simulink library "xps_library"  (Simulink 6.2)
values from neighbouring files (symbols this model uses):
  BEE2_ctrl =     [BEE2_hw_routes.mat]
  CORR =     [BEE2_hw_routes.mat]
  iBOB =     [BEE2_hw_routes.mat]
  out = 0    [read_xps.m]    (also in write_xps.m)
undefined symbols (not defined in the file or in its folder): powerpc405, xps_library_software_register_user_data_in
libraries: xbsIndex_r3 x302, simulink x29, dspsigops x12, xps_library x6
(part 1 of 3)
settings Model: LastModifiedBy=hchen05

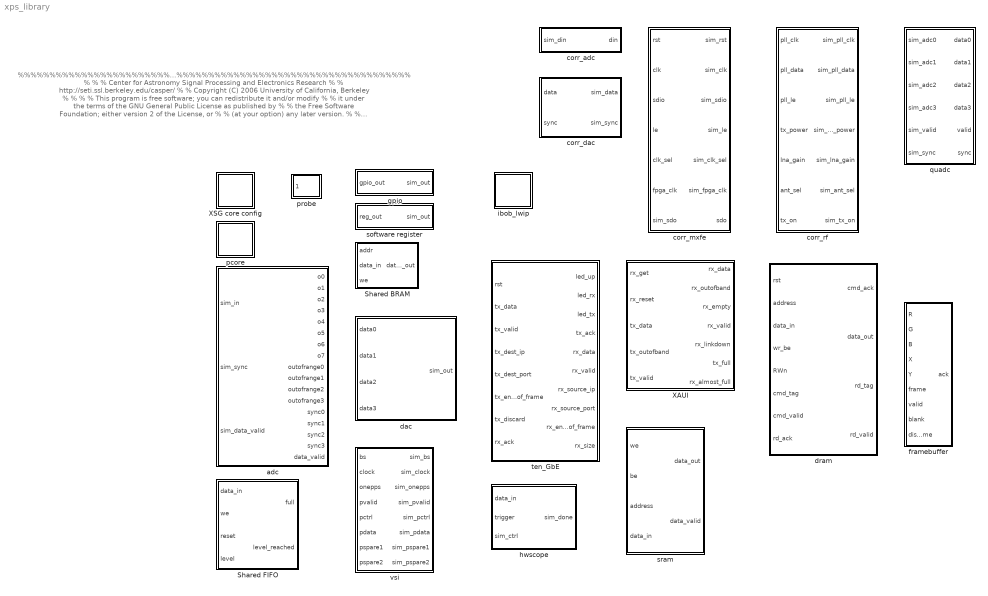
== system xps_library ==
  note: %%%%%%%%%%%%%%%%%%%%%%%%%%%%%%%%%%%%%%%%%%%%%%%%%%%%%%%%%%%%%%%%%%%%%%%%%%%%%%%
      | %                                                                             %
      | %   Center for Astronomy Signal Processing and Electronics Research           %
      | %   http://seti.ssl.berkeley.edu/casper/                                      %
      | %   Copyright (C) 2006 University of California, Berkeley                     %
      | %                                                                             %
      | %   This program is free software; you can redistribute it and/or modify      %
      | %   it under the terms of the GNU General Public License as published by      %
      | %   the Free Software Foundation; either version 2 of the License, or         %
      | %   (at your option) any later version.                                       %
      | %                                                                             %
      | %   This program is distributed in the hope that it will be useful,           %
      | %   but WITHOUT ANY WARRANTY; without even the implied warranty of            %
      | %   MERCHANTABILITY or FITNESS FOR A PARTICULAR PURPOSE.  See the             %
      | %   GNU General Public License for more details.                              %
      | %                                                                             %
      | %   You should have received a copy of the GNU General Public License along   %
      | %   with this program; if not, write to the Free Software Foundation, Inc.,   %
      | %   51 Franklin Street, Fifth Floor, Boston, MA 02110-1301 USA.               %
      | %                                                                             %
      | %%%%%%%%%%%%%%%%%%%%%%%%%%%%%%%%%%%%%%%%%%%%%%%%%%%%%%%%%%%%%%%%%%%%%%%%%%%%%%%
  Shared BRAM : Subsystem  Tag=xps:bram  mask{arith_type=Signed  (2's comp), addr_width=11, data_width=32, data_bin_pt=0, init_vals=[1:2^11], sample_rate=1}
      mask prompts: arith_type "Output Data Type"; addr_width "Address width"; data_width "Data Width"; data_bin_pt "Data Binary Point"; init_vals "Initial values (simulation only)"; sample_rate "Sample rate"
      mask init:
      | shared_bram_mask;
      mask StyleString: popup(Unsigned|Signed  (2's comp)),edit,edit,edit,edit,edit
  Shared FIFO : Subsystem  Tag=xps:fifo  mask{io_dir=To Processor, arith_type=Unsigned, data_width=32, data_bin_pt=0, fifo_length=512}
      mask prompts: io_dir "I/O Direction:"; arith_type "Data Type:"; data_width "Data Width:"; data_bin_pt "Data Binary Point:"; fifo_length "Depth:"
      mask init:
      | fifo_mask;
      mask StyleString: popup(From Processor|To Processor),popup(Unsigned|Signed  (2's comp)),popup(4|8|16|32|64|128|256),edit,popup(512|1024|2048|4096|8192|16384|32768|65536)
  XAUI : Subsystem  Tag=xps:xaui  mask(xaui){demux=1, port=iBOB:0, show_param=off, pre_emph=3, swing=800}
      mask prompts: show_param "---------------------- Show Implementation Parameters -----------------------------------------------------------------------------------"; pre_emph "Pre-emphasis"; swing "Differential swing"
      mask help: XAUI block for sending and receiving point-to-point, streaming data over the BEE2 and iBOB's CX4 connectors. NOTE: A new version of this block is in development.
      mask init:
      | xaui_mask;
      mask Help: eval('xlWeb([getenv(''MLIB_ROOT''), ''\doc\html\com_xaui\com_xaui.html''])')
      mask StyleString: popup(1|2),popup(iBOB:0|iBOB:1|BEE2_ctrl:0|BEE2_ctrl:1|BEE2_usr:0|BEE2_usr:1|BEE2_usr:2|BEE2_usr:3|CORR:0),checkbox,popup(0|1|2|3),popup(400|500|600|700|800)
      mask CallbackString:
      | ||myname=gcb;
      | if strcmp(get_param(myname, 'show_param'), 'on')
      |     set_param(myname, 'MaskVisibilities', {'on','on','on','on','on'});
      | else
      |     set_param(myname, 'MaskVisibilities', {'on','on','on','off','off'});
      | end||
  XSG core config : Subsystem  Tag=xps:xsg  mask(xsg core config){hw_sys=iBOB, ibob_linux=off, clk_src=sys_clk, gpio_clk_io_group=iBOB:sma, gpio_clk_bit_index=0, clk_rate=100, sample_period=1, synthesis_tool=XST, mpc_type=powerpc405}
      mask prompts: hw_sys "Hardware Platform"; ibob_linux "Include Linux add-on board support"; clk_src "User IP Clock source"; gpio_clk_io_group "GPIO Clock Pin I/O group"; gpio_clk_bit_index "GPIO Clock Pin bit index"; clk_rate "User IP Clock Rate (MHz)"; sample_period "Sample Period"; synthesis_tool "Synthesis Tool:"; mpc_type "Mask Parameter 10:"
      mask help:
      | The XSG Core Config block is used to configure the System Generator design
      | for the bee_xps toolflow. Settings here are used to configure the
      | Xilinx System Generator block parameters automatically, and control toolflow
      | script  execution. It needs to be at the top level of all designs being compiled
      | with the bee_xps toolflow.
      mask init:
      | xps_xsg_conf_mask;
      mask Help: eval('xlWeb([getenv(''MLIB_ROOT''), ''\doc\html\sys_xsg_core_config\sys_xsg_core_config.html''])')
      mask StyleString: popup(iBOB|BEE2_ctrl|BEE2_usr|CORR),checkbox,popup(sys_clk|sys_clk2x|usr_clk|usr_clk2x|adc0_clk|adc1_clk|dac0_clk|dac1_clk),popup(iBOB:gpio0|iBOB:gpio1|iBOB:gpio2|iBOB:gpio3|iBOB:sma|iBOB:zdok0|iBOB:zdok1|iBOB:mdr),edit,edit,edit,popup(Leonardo Spectrum|Synplify|Synplify Pro|XST),edit
      mask CallbackString:
      | myname=gcb;
      | if strcmp(get_param(myname,'hw_sys'), 'iBOB')
      |     if strmatch('usr_clk', get_param(myname,'clk_src'))
      |         set_param(myname, 'MaskVisibilities', {'on','on','on','on','on','on','on','on','off'});
      |     else
      |         set_param(myname, 'MaskVisibilities', {'on','on','on','off','off','on','on','on','off'});
      |     end
      | else
      |     set_param(myname, 'MaskVisibilities', {'on','off','on','off','off','on','on','on','off'});
      | end||myname=gcb;
      | if strcmp(get_param(myname,'hw_sys'), 'iBOB')
      |     if strmatch('usr_clk', get_param(myname,'clk_src'))
      |         set_param(myname, 'MaskVisibilities', {'on','on','on','on','on','on','on','on','off'});
      |     else
      |         set_param(myname, 'MaskVisibilities', {'on','on','on','off','off','on','on','on','off'});
      |     end
      | else
      |     set_param(myname, 'MaskVisibilities', {'on','off','on','off','off','on','on','on','off'});
      | end||||||
      mask Display: fprintf('MSSGE');
  adc : Subsystem  Tag=xps:adc  mask(adc){adc_brd=iBOB:adc0, adc_clk_rate=800, adc_interleave=on, sample_period=1}
      mask prompts: adc_brd "ADC board"; adc_clk_rate "ADC clock rate (MHz)"; adc_interleave "ADC interleave mode"; sample_period "Sample period"
      mask help: The ADC block converts analog inputs to digital outputs. Every clock cycle, the inputs are sampled and digitized to 8 bit binary point numbers in the range of [-1, 1) and are then output by the adc.
      mask init:
      | adc_mask;
      mask Help: eval('xlWeb([getenv(''MLIB_ROOT''), ''\doc\html\sys_adc\sys_adc.html''])')
      mask StyleString: popup(iBOB:adc0|iBOB:adc1),edit,checkbox,edit
  corr_adc : Subsystem  Tag=xps:corr_adc  mask{adc_brd=CORR:adc_i, arith_type=Signed  (2's comp), data_bin_pt=11, reg_clk_phase=0, sample_period=1}
      mask prompts: adc_brd "ADC:"; arith_type "Data type:"; data_bin_pt "Binary point:"; reg_clk_phase "Input sample clock phase:"; sample_period "Sample period:"
      mask init:
      | corr_adc_mask;
      mask StyleString: popup(CORR:adc_i|CORR:adc_q),popup(Unsigned|Signed  (2's comp)),edit,popup(0|90|180|270),edit
  corr_dac : Subsystem  Tag=xps:corr_dac  mask{arith_type=Unsigned, bin_pt=12, reg_clk_phase=0, sample_period=1}
      mask prompts: arith_type "Data Type:"; bin_pt "Data binary point (14-bit data):"; reg_clk_phase "Output sample clock phase:"; sample_period "Sample period:"
      mask init:
      | corr_dac_mask;
      mask StyleString: popup(Boolean|Unsigned|Signed  (2's comp)),edit,popup(0|90|180|270),edit
  corr_mxfe : Subsystem  Tag=xps:corr_mxfe  mask{reg_clk_phase=0, sample_period=1}
      mask prompts: reg_clk_phase "Input sample clock phase:"; sample_period "Sample period:"
      mask init:
      | corr_mxfe_mask;
      mask StyleString: popup(0|90|180|270),edit
  corr_rf : Subsystem  Tag=xps:corr_rf  mask{arith_type=Unsigned, bin_pt=0, sample_period=1}
      mask prompts: arith_type "TX power data type:"; bin_pt "TX power binary point (3-bit data):"; sample_period "Sample period:"
      mask init:
      | corr_rf_mask;
      mask StyleString: popup(Boolean|Unsigned|Signed  (2's comp)),edit,edit
  dac : Subsystem  Tag=xps:dac  mask(dac){dac_brd=iBOB:dac0, dac_clk_rate=800, sample_period=1, show_param=off, invert_clock=off}
      mask prompts: dac_brd "DAC board"; dac_clk_rate "DAC clock rate (MHz)"; sample_period "Sample period"; show_param "---------------------- Show Implementation Parameters -----------------------------------------------------------------------------------"; invert_clock "Invert output clock phase"
      mask help: Interface to SiBeam single Atmel TS86101G2B DAC board. The DAC block converts 4 digital inputs to 1 analog output. The dac runs at 4x FPGA clock frequency, outputting analog converted samples 0 through 3 each FPGA clock cycle.
      mask init:
      | dac_mask;
      mask Help: eval('xlWeb([getenv(''MLIB_ROOT''), ''\doc\html\sys_dac\sys_dac.html''])')
      mask StyleString: popup(iBOB:dac0|iBOB:dac1),edit,edit,checkbox,checkbox
      mask CallbackString:
      | |||myname=gcb;
      | if strcmp(get_param(myname, 'show_param'), 'on')
      |     set_param(myname, 'MaskVisibilities', {'on','on','on','on','on'});
      | else
      |     set_param(myname, 'MaskVisibilities', {'on','on','on','on','off'});
      | end|
  dram : Subsystem  Tag=xps:dram  mask(dram){dimm=1, arith_type=Unsigned, bin_pt=0, ip_clock=200, sample_period=1, use_sim=on, bank_mgt=off, wide_data=off, half_burst=off}
      mask prompts: arith_type "Data Type"; bin_pt "Data binary point"; ip_clock "Datapath clock rate (MHz)"; sample_period "Sample period"; use_sim "Simulate DRAM using ModelSim"; bank_mgt "Enable bank management"; wide_data "Use wide data bus (288 bits)"; half_burst "Use half-burst"
      mask help:
      | Interface to 1GB DDR2 DIMMs on BEE2.
      |
      | To simulate using ModelSim, place a ModelSim block named 'ModelSim' (case-sensitive) in the top level of the design.
      |
      | Commands that are clocked-in are executed with an unknown delay, however, execution order is maintained.
      mask init:
      | dram_mask;
      mask Help: eval('xlWeb([getenv(''MLIB_ROOT''), ''\doc\html\sys_dram\sys_dram.html''])')
      mask StyleString: popup(1|2|3|4),popup(Boolean|Unsigned|Signed  (2's comp)),edit,edit,edit,checkbox,checkbox,checkbox,checkbox
      mask CallbackString:
      | |||||||myname=gcb;
      | if strcmp(get_param(myname, 'wide_data'), 'off')
      |     set_param(myname, 'MaskEnables', {'on','on','on','on','on','on','on','on','on'});
      | else
      |     set_param(myname, 'half_burst', 'off');
      |     set_param(myname, 'MaskEnables', {'on','on','on','on','on','on','on','on','off'});
      | end|
  framebuffer : Subsystem  Tag=xps:framebuffer  mask(framebuffer){dimm=2, sample_period=1}
      mask prompts: sample_period "Sample period"
      mask help: Interface to Framebuffer.
      mask init:
      | framebuffer_mask;
      mask StyleString: popup(2|3|4),edit
  gpio : Subsystem  Tag=xps:gpio  mask(gpio){io_group=iBOB:led, io_dir=out, arith_type=Boolean, bitwidth=1, bin_pt=0, bit_index=0, sample_period=1, use_single_ended=off, use_ddr=off, reg_iob=on, reg_clk_phase=0, termination=None}
      mask prompts: io_group "I/O group"; io_dir "I/O direction"; arith_type "Data Type"; bitwidth "Data bitwidth"; bin_pt "Data binary point"; bit_index "GPIO bit index"; sample_period "Sample period"; use_single_ended "Use as single-ended"; use_ddr "Use DDR"; reg_iob "Pack register in the pad"; reg_clk_phase "Register clock phase"; termination "Termination method"
      mask help: GPIO interfaces for BEE2, iBOB, and CORR boards.
      mask init:
      | gpio_mask;
      mask StyleString: popup(iBOB:led|iBOB:dipsw|iBOB:gpio0|iBOB:gpio1|iBOB:gpio2|iBOB:gpio3|iBOB:zdok0|iBOB:zdok1|iBOB:mdr|iBOB:sma|BEE2_ctrl:led|BEE2_ctrl:downlink1|BEE2_ctrl:downlink2|BEE2_ctrl:downlink3|BEE2_ctrl:downlink4|BEE2_usr:led|BEE2_usr:gpio|BEE2_usr:bus_ctrl|BEE2_usr:bus_data|BEE2_usr:uplink|BEE2_usr:leftlink|BEE2_usr:rightlink|CORR:four_buttons|CORR:six_buttons|CORR:led|CORR:jumper_driver|CORR:jumper_receiver),popup(in|out),popup(Boolean|Unsigned|Signed  (2's comp)),edit,edit,edit,edit,checkbox,checkbox,checkbox,popup(0|90|180|270),popup(None|Pullup|Pulldown)
      mask CallbackString:
      | if ~isempty(find(strcmp(get_param(gcb, 'io_group'), {'iBOB:zdok0' 'iBOB:zdok1' 'iBOB:mdr'})))
      |     set_param(gcb, 'MaskVisibilities', {'on','on','on','on','on','on','on','on','on','on','on','on'});
      | else
      |     set_param(gcb, 'MaskVisibilities', {'on','on','on','on','on','on','on','off','on','on','on','on'});
      | end|||||||if ~isempty(find(strcmp(get_param(gcb,'io_group'),{'iBOB:zdok0','iBOB:zdok1','iBOB:mdr'}))) & strcmp(get_param(gcb,'use_single_ended'),'on')
      |     warndlg('The selected I/O group is routed as a differential pair on the board. Using these I/Os in single-ended mode may degrade signal integrity performance.')
      | end|if strcmp(get_param(gcb,'use_ddr'),'on')
      |     set_param(gcb,'reg_iob','on');
      | end|||
  hwscope : Subsystem  mask{scope_depth=2048, sim_trig_delay=8}
      mask prompts: scope_depth "Scope depth:"; sim_trig_delay "Trigger delay (simulation only):"
      mask init:
      | cursys = gcb;
      | set_param([cursys,'/scopefifo'], 'fifo_length', scope_depth);
      mask StyleString: popup(512|1024|2048|4096|8192|16384|32768|65536),edit
  ibob_lwip : Subsystem
      mask Type: ibobethlite
      mask Description: Attaches SRAM0 to the PLB bus and adds LWIP support.
      mask Display: fprintf('IBOB\nLWIP');
  pcore : Subsystem  Tag=xps:pcore  mask(pcore){pcore_path=customlib/pcores}
      mask prompts: pcore_path "Custom pcores path"
      mask help: Allows insertion of custom EDK pcores not distributed with base systems.
      mask Display: fprintf('PCORE');
  probe : Subsystem  Tag=xps:probe  mask{ila_number=0, match_type=basic, match_counter_width=8, capture_depth=512, arith_type=Boolean, bitwidth=1, bin_pt=0}
      mask prompts: ila_number "Chipscope ILA number"; match_type "Match Unit Type"; match_counter_width "Match counter width"; capture_depth "Probe capture depth"; arith_type "Data type"; bitwidth "Data bit width"; bin_pt "Data binary point"
      mask init:
      | probe_mask;
      mask StyleString: popup(0|1|2|3|4|5|6|7|8|9|10|11|12|13|14),popup(basic|basic with edges|extended|extended with edges|range|range with edges),popup(0|8|16|24|32),popup(512|1024|2048|4096|8192|16384),popup(Boolean|Unsigned|Signed  (2's comp)),edit,edit
  quadc : Subsystem  Tag=xps:quadc  mask(CASPER QuADC Interface Block){adc_brd=0, adc_clk_rate=200}
      mask prompts: adc_brd "ADC Board"; adc_clk_rate "ADC Clock Rate (MHz)"
      mask help: Interface block for the CASPER Quad ADC board (ADC4x250-8).
      mask init:
      | quadc_mask;
      mask StyleString: popup(0|1),edit
  software register : Subsystem  Tag=xps:sw_reg  mask{io_dir=To Processor, arith_type=Unsigned, bitwidth=32, bin_pt=0, sample_period=1, gw_name=xps_library_software_register_user_data_in}
      mask prompts: io_dir "I/O direction"; arith_type "Data Type"; bitwidth "Data bitwidth"; bin_pt "Data binary point"; sample_period "Sample period"; gw_name "Mask Parameter 6:"
      mask init:
      | register_mask;
      mask StyleString: popup(From Processor|To Processor),popup(Unsigned|Signed  (2's comp)),edit,edit,edit,edit
  sram : Subsystem  Tag=xps:sram  mask(sram){sram=0, arith_type=Unsigned, bin_pt=0, sample_period=1, use_sim=off}
      mask prompts: arith_type "Data Type"; bin_pt "Data binary point (bitwidth is 36)"; sample_period "Sample period"; use_sim "Simulate SRAM using ModelSim"
      mask help:
      | Interface to CY7C1370DV25 36x512k SRAMs on IBOB.
      |
      | To simulate using ModelSim, place a ModelSim block named 'ModelSim' (case-sensitive) in the top level of the design.
      |
      | The sram block represents a 36x512k SRAM chip on the IBOB. It stores 36-bit words and requires 19 bits to access its address space.
      mask init:
      | sram_mask;
      mask Help: eval('xlWeb([getenv(''MLIB_ROOT''), ''\doc\html\sys_sram\sys_sram.html''])')
      mask StyleString: popup(0|1),popup(Boolean|Unsigned|Signed  (2's comp)),edit,edit,checkbox
  ten_GbE : Subsystem  Tag=xps:tengbe  mask(ten_GbE){port=BEE2_ctrl:0, mac_lite=off, show_param=off, pre_emph=3, swing=800}
      mask prompts: mac_lite "Use light-weight MAC: Warning --> it DOES NOT check any CRC on receive"; show_param "---------------------- Show Implementation Parameters -----------------------------------------------------------------------------------"; pre_emph "Pre-emphasis"; swing "Differential swing"
      mask help: This block sends and receives UDP frames (packets). It accepts a 64 bit wide data stream with user-determined frame breaks. The data stream is wrapped in a UDP frame for transmission. Incoming UDP packets are unwrapped and the data presented as a 64 bit wide stream.
      mask init:
      | tengbe_mask;
      mask Help: eval('xlWeb([getenv(''MLIB_ROOT''), ''\doc\html\com_ten_GbE\com_ten_GbE.html''])')
      mask StyleString: popup(iBOB:0|iBOB:1|BEE2_ctrl:0|BEE2_ctrl:1|BEE2_usr:0|BEE2_usr:1|BEE2_usr:2|BEE2_usr:3|CORR:0),checkbox,checkbox,popup(0|1|2|3),popup(400|500|600|700|800)
      mask CallbackString:
      | ||myname=gcb;
      | if strcmp(get_param(myname, 'show_param'), 'on')
      |     set_param(myname, 'MaskVisibilities', {'on','on','on','on', 'on'});
      | else
      |     set_param(myname, 'MaskVisibilities', {'on','on','on','off','off'});
      | end||
  vsi : Subsystem  Tag=xps:vsi  mask(vsi){connector=MDR, arith_type=Unsigned, bin_pt=0, sample_period=1}
      mask prompts: arith_type "Data Type"; bin_pt "Data binary point (bitwidth is 32)"; sample_period "Sample period"
      mask help: Interface to MDR-80 connector on IBOB as configured for VLBI Standard Interface.
      mask init:
      | vsi_mask;
      mask StyleString: popup(MDR|ZDOK 1),popup(Boolean|Unsigned|Signed  (2's comp)),edit,edit

== system xps_library/Shared BRAM ==
  addr : Inport  Port=1  LatchInput=off
  data_in : Inport  Port=2  LatchInput=off
  we : Inport  Port=3  LatchInput=off
  Convert : xbsIndex_r3/Convert  arith_type=Unsigned  n_bits=addr_width  bin_pt=0  quantization=Truncate  overflow=Wrap  latency=0  explicit_period=off  period=1  dbl_ovrd=off  show_param=off  inserted_by_tool=off  pipeline=off
      settings: xl_area=[0, 0, 0, 0, 0, 0, 0]
  Convert1 : xbsIndex_r3/Convert  arith_type=Unsigned  n_bits=1  bin_pt=0  quantization=Truncate  overflow=Wrap  latency=0  explicit_period=off  period=1  dbl_ovrd=off  show_param=off  inserted_by_tool=off  pipeline=off
      settings: xl_area=[0, 0, 0, 0, 0, 0, 0]
  Convert2 : xbsIndex_r3/Convert  arith_type="Signed  (2's comp)"  n_bits=data_width  bin_pt=data_bin_pt  quantization=Truncate  overflow=Wrap  latency=0  explicit_period=off  period=1  dbl_ovrd=off  show_param=off  inserted_by_tool=off  pipeline=off
      settings: xl_area=[0, 0, 0, 0, 0, 0, 0]
  mem : Subsystem
  xps_library_Shared_BRAM_addr : xbsIndex_r3/Gateway Out  output_type=Double  nbits=8  bin_pt=6  arith_type=Boolean  quantization=Truncate  overflow=Wrap  hdl_port=on  timing_constraint=None  locs_specified=off  LOCs={'A5','B9','A9','C1','A3','G6','E9','A6','A7','A8','B8','B1','B3','D9','B5','B4','B6','C2'}  needs_fixed_name=on  show_param=off
      settings: xl_area=[0, 0, 0, 0, 0, 0, 0]
  xps_library_Shared_BRAM_data_in : xbsIndex_r3/Gateway Out  output_type=Double  nbits=8  bin_pt=6  arith_type=Boolean  quantization=Truncate  overflow=Wrap  hdl_port=on  timing_constraint=None  locs_specified=off  LOCs={'B21','B22','A22','B23','B19','C19','A20','A21','A23','B24','A24','A25','E18','D18','C18','B18'}  needs_fixed_name=on  show_param=off
      settings: xl_area=[0, 0, 0, 0, 0, 0, 0]
  xps_library_Shared_BRAM_data_out : xbsIndex_r3/Gateway In  arith_type="Signed  (2's comp)"  n_bits=data_width  bin_pt=data_bin_pt  quantization=Truncate  overflow=Wrap  period=sample_rate  timing_constraint=None  locs_specified=off  LOCs={}  needs_fixed_name=on  dbl_ovrd=off  show_param=off
      settings: xl_area=[0, 0, 0, 0, 0, 0, 0]
  xps_library_Shared_BRAM_we : xbsIndex_r3/Gateway Out  output_type=Double  nbits=8  bin_pt=6  arith_type=Boolean  quantization=Truncate  overflow=Wrap  hdl_port=on  timing_constraint=None  locs_specified=off  LOCs={'A14'}  needs_fixed_name=on  show_param=off
      settings: xl_area=[0, 0, 0, 0, 0, 0, 0]
  data_out : Outport
  wires:
  mem/1(Out1) -> xps_library_Shared_BRAM_data_out/1
  data_in/1 -> Convert2/1
  xps_library_Shared_BRAM_data_out/1 -> data_out/1
  addr/1 -> Convert/1
  we/1 -> Convert1/1
  Convert/1 -> xps_library_Shared_BRAM_addr/1
  Convert1/1 -> xps_library_Shared_BRAM_we/1
  Convert2/1 -> xps_library_Shared_BRAM_data_in/1
  xps_library_Shared_BRAM_addr/1 -> mem/1(In1)
  xps_library_Shared_BRAM_data_in/1 -> mem/2(In2)
  xps_library_Shared_BRAM_we/1 -> mem/3(In3)

== system xps_library/Shared FIFO ==
  data_in : Inport  Port=1  LatchInput=off
  we : Inport  Port=2  LatchInput=off
  reset : Inport  Port=3  LatchInput=off
  level : Inport  Port=4  LatchInput=off
  convert_xps_library_Shared_FIFO_user_data_in : xbsIndex_r3/Convert  arith_type=Unsigned  n_bits=32  bin_pt=0  quantization=Truncate  overflow=Wrap  latency=0  explicit_period=off  period=1  dbl_ovrd=off  show_param=off  inserted_by_tool=off  pipeline=off
      settings: xl_area=[0, 0, 0, 0, 0, 0, 0]
  convert_xps_library_Shared_FIFO_user_level : xbsIndex_r3/Convert  arith_type=Unsigned  n_bits=16  bin_pt=0  quantization=Truncate  overflow=Wrap  latency=0  explicit_period=off  period=1  dbl_ovrd=off  show_param=off  inserted_by_tool=off  pipeline=off
      settings: xl_area=[0, 0, 0, 0, 0, 0, 0]
  convert_xps_library_Shared_FIFO_user_reset : xbsIndex_r3/Convert  arith_type=Unsigned  n_bits=1  bin_pt=0  quantization=Truncate  overflow=Wrap  latency=0  explicit_period=off  period=1  dbl_ovrd=off  show_param=off  inserted_by_tool=off  pipeline=off
      settings: xl_area=[0, 0, 0, 0, 0, 0, 0]
  convert_xps_library_Shared_FIFO_user_we : xbsIndex_r3/Convert  arith_type=Unsigned  n_bits=1  bin_pt=0  quantization=Truncate  overflow=Wrap  latency=0  explicit_period=off  period=1  dbl_ovrd=off  show_param=off  inserted_by_tool=off  pipeline=off
      settings: xl_area=[0, 0, 0, 0, 0, 0, 0]
  xps_library_Shared_FIFO_user_data_in : xbsIndex_r3/Gateway Out  output_type=Double  nbits=8  bin_pt=6  arith_type=Boolean  quantization=Truncate  overflow=Wrap  hdl_port=on  timing_constraint=None  locs_specified=off  LOCs={}  needs_fixed_name=off  show_param=off
      settings: xl_area=[0, 0, 0, 0, 0, 0, 0]
  xps_library_Shared_FIFO_user_full : xbsIndex_r3/Gateway In  arith_type=Boolean  n_bits=1  bin_pt=0  quantization=Truncate  overflow=Wrap  period=1  timing_constraint=None  locs_specified=off  LOCs={}  needs_fixed_name=off  dbl_ovrd=off  show_param=off
      settings: xl_area=[0, 0, 0, 0, 0, 0, 0]
  xps_library_Shared_FIFO_user_level : xbsIndex_r3/Gateway Out  output_type=Double  nbits=8  bin_pt=6  arith_type=Boolean  quantization=Truncate  overflow=Wrap  hdl_port=on  timing_constraint=None  locs_specified=off  LOCs={}  needs_fixed_name=off  show_param=off
      settings: xl_area=[0, 0, 0, 0, 0, 0, 0]
  xps_library_Shared_FIFO_user_level_reached : xbsIndex_r3/Gateway In  arith_type=Boolean  n_bits=1  bin_pt=0  quantization=Truncate  overflow=Wrap  period=1  timing_constraint=None  locs_specified=off  LOCs={}  needs_fixed_name=off  dbl_ovrd=off  show_param=off
      settings: xl_area=[0, 0, 0, 0, 0, 0, 0]
  xps_library_Shared_FIFO_user_reset : xbsIndex_r3/Gateway Out  output_type=Double  nbits=8  bin_pt=6  arith_type=Boolean  quantization=Truncate  overflow=Wrap  hdl_port=on  timing_constraint=None  locs_specified=off  LOCs={}  needs_fixed_name=off  show_param=off
      settings: xl_area=[0, 0, 0, 0, 0, 0, 0]
  xps_library_Shared_FIFO_user_we : xbsIndex_r3/Gateway Out  output_type=Double  nbits=8  bin_pt=6  arith_type=Boolean  quantization=Truncate  overflow=Wrap  hdl_port=on  timing_constraint=None  locs_specified=off  LOCs={}  needs_fixed_name=off  show_param=off
      settings: xl_area=[0, 0, 0, 0, 0, 0, 0]
  full : Outport
  level_reached : Outport  Port=2
  wires:
  data_in/1 -> convert_xps_library_Shared_FIFO_user_data_in/1
  convert_xps_library_Shared_FIFO_user_data_in/1 -> xps_library_Shared_FIFO_user_data_in/1
  we/1 -> convert_xps_library_Shared_FIFO_user_we/1
  convert_xps_library_Shared_FIFO_user_we/1 -> xps_library_Shared_FIFO_user_we/1
  reset/1 -> convert_xps_library_Shared_FIFO_user_reset/1
  convert_xps_library_Shared_FIFO_user_reset/1 -> xps_library_Shared_FIFO_user_reset/1
  level/1 -> convert_xps_library_Shared_FIFO_user_level/1
  convert_xps_library_Shared_FIFO_user_level/1 -> xps_library_Shared_FIFO_user_level/1
  xps_library_Shared_FIFO_user_full/1 -> full/1
  xps_library_Shared_FIFO_user_level_reached/1 -> level_reached/1

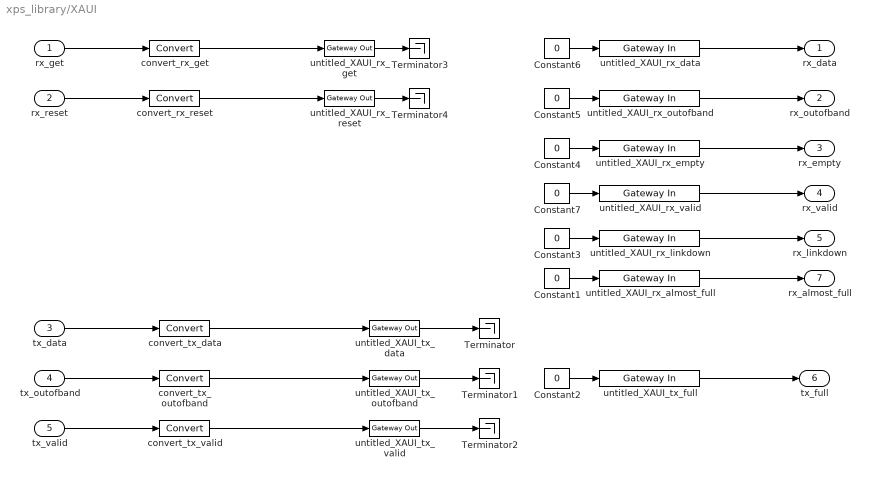
== system xps_library/XAUI ==
  rx_get : Inport  Port=1  LatchInput=off
  rx_reset : Inport  Port=2  LatchInput=off
  tx_data : Inport  Port=3  LatchInput=off
  tx_outofband : Inport  Port=4  LatchInput=off
  tx_valid : Inport  Port=5  LatchInput=off
  Constant{1..7} (7 alike) : Constant  Value=0
  Terminator{,1..4} (5 alike) : Terminator
  convert_rx_get : xbsIndex_r3/Convert  arith_type=Boolean  n_bits=64  bin_pt=0  quantization=Truncate  overflow=Wrap  latency=0  explicit_period=off  period=1  dbl_ovrd=off  show_param=off  inserted_by_tool=off  pipeline=off
      settings: xl_area=[0, 0, 0, 0, 0, 0, 0]
  convert_rx_reset : xbsIndex_r3/Convert  arith_type=Boolean  n_bits=1  bin_pt=0  quantization=Truncate  overflow=Wrap  latency=0  explicit_period=off  period=1  dbl_ovrd=off  show_param=off  inserted_by_tool=off  pipeline=off
      settings: xl_area=[0, 0, 0, 0, 0, 0, 0]
  convert_tx_data : xbsIndex_r3/Convert  arith_type=Unsigned  n_bits=64  bin_pt=0  quantization=Truncate  overflow=Wrap  latency=0  explicit_period=off  period=1  dbl_ovrd=off  show_param=off  inserted_by_tool=off  pipeline=off
      settings: xl_area=[0, 0, 0, 0, 0, 0, 0]
  convert_tx_outofband : xbsIndex_r3/Convert  arith_type=Unsigned  n_bits=8  bin_pt=0  quantization=Truncate  overflow=Wrap  latency=0  explicit_period=off  period=1  dbl_ovrd=off  show_param=off  inserted_by_tool=off  pipeline=off
      settings: xl_area=[0, 0, 0, 0, 0, 0, 0]
  convert_tx_valid : xbsIndex_r3/Convert  arith_type=Boolean  n_bits=1  bin_pt=0  quantization=Truncate  overflow=Wrap  latency=0  explicit_period=off  period=1  dbl_ovrd=off  show_param=off  inserted_by_tool=off  pipeline=off
      settings: xl_area=[0, 0, 0, 0, 0, 0, 0]
  untitled_XAUI_rx_almost_full : xbsIndex_r3/Gateway In  arith_type=Boolean  n_bits=1  bin_pt=0  quantization=Truncate  overflow=Wrap  period=1  timing_constraint=None  locs_specified=off  LOCs={}  needs_fixed_name=off  dbl_ovrd=off  show_param=off
      settings: xl_area=[0, 0, 0, 0, 0, 0, 0]
  untitled_XAUI_rx_data : xbsIndex_r3/Gateway In  arith_type=Unsigned  n_bits=64  bin_pt=0  quantization=Truncate  overflow=Wrap  period=1  timing_constraint=None  locs_specified=off  LOCs={}  needs_fixed_name=off  dbl_ovrd=off  show_param=off
      settings: xl_area=[0, 0, 0, 0, 0, 0, 0]
  untitled_XAUI_rx_empty : xbsIndex_r3/Gateway In  arith_type=Boolean  n_bits=1  bin_pt=0  quantization=Truncate  overflow=Wrap  period=1  timing_constraint=None  locs_specified=off  LOCs={}  needs_fixed_name=off  dbl_ovrd=off  show_param=off
      settings: xl_area=[0, 0, 0, 0, 0, 0, 0]
  untitled_XAUI_rx_get : xbsIndex_r3/Gateway Out  output_type=Double  nbits=8  bin_pt=6  arith_type=Boolean  quantization=Truncate  overflow=Wrap  hdl_port=on  timing_constraint=None  locs_specified=off  LOCs={}  needs_fixed_name=off  show_param=off
      settings: xl_area=[0, 0, 0, 0, 0, 0, 0]
  untitled_XAUI_rx_linkdown : xbsIndex_r3/Gateway In  arith_type=Boolean  n_bits=1  bin_pt=0  quantization=Truncate  overflow=Wrap  period=1  timing_constraint=None  locs_specified=off  LOCs={}  needs_fixed_name=off  dbl_ovrd=off  show_param=off
      settings: xl_area=[0, 0, 0, 0, 0, 0, 0]
  untitled_XAUI_rx_outofband : xbsIndex_r3/Gateway In  arith_type=Unsigned  n_bits=8  bin_pt=0  quantization=Truncate  overflow=Wrap  period=1  timing_constraint=None  locs_specified=off  LOCs={}  needs_fixed_name=off  dbl_ovrd=off  show_param=off
      settings: xl_area=[0, 0, 0, 0, 0, 0, 0]
  untitled_XAUI_rx_reset : xbsIndex_r3/Gateway Out  output_type=Double  nbits=8  bin_pt=6  arith_type=Boolean  quantization=Truncate  overflow=Wrap  hdl_port=on  timing_constraint=None  locs_specified=off  LOCs={}  needs_fixed_name=off  show_param=off
      settings: xl_area=[0, 0, 0, 0, 0, 0, 0]
  untitled_XAUI_rx_valid : xbsIndex_r3/Gateway In  arith_type=Boolean  n_bits=1  bin_pt=0  quantization=Truncate  overflow=Wrap  period=1  timing_constraint=None  locs_specified=off  LOCs={}  needs_fixed_name=off  dbl_ovrd=off  show_param=off
      settings: xl_area=[0, 0, 0, 0, 0, 0, 0]
  untitled_XAUI_tx_data : xbsIndex_r3/Gateway Out  output_type=Double  nbits=8  bin_pt=6  arith_type=Boolean  quantization=Truncate  overflow=Wrap  hdl_port=on  timing_constraint=None  locs_specified=off  LOCs={}  needs_fixed_name=off  show_param=off
      settings: xl_area=[0, 0, 0, 0, 0, 0, 0]
  untitled_XAUI_tx_full : xbsIndex_r3/Gateway In  arith_type=Boolean  n_bits=1  bin_pt=0  quantization=Truncate  overflow=Wrap  period=1  timing_constraint=None  locs_specified=off  LOCs={}  needs_fixed_name=off  dbl_ovrd=off  show_param=off
      settings: xl_area=[0, 0, 0, 0, 0, 0, 0]
  untitled_XAUI_tx_outofband : xbsIndex_r3/Gateway Out  output_type=Double  nbits=8  bin_pt=6  arith_type=Boolean  quantization=Truncate  overflow=Wrap  hdl_port=on  timing_constraint=None  locs_specified=off  LOCs={}  needs_fixed_name=off  show_param=off
      settings: xl_area=[0, 0, 0, 0, 0, 0, 0]
  untitled_XAUI_tx_valid : xbsIndex_r3/Gateway Out  output_type=Double  nbits=8  bin_pt=6  arith_type=Boolean  quantization=Truncate  overflow=Wrap  hdl_port=on  timing_constraint=None  locs_specified=off  LOCs={}  needs_fixed_name=off  show_param=off
      settings: xl_area=[0, 0, 0, 0, 0, 0, 0]
  rx_data : Outport
  rx_outofband : Outport  Port=2
  rx_empty : Outport  Port=3
  rx_valid : Outport  Port=4
  rx_linkdown : Outport  Port=5
  tx_full : Outport  Port=6
  rx_almost_full : Outport  Port=7
  wires:
  rx_get/1 -> convert_rx_get/1
  convert_rx_get/1 -> untitled_XAUI_rx_get/1
  rx_reset/1 -> convert_rx_reset/1
  convert_rx_reset/1 -> untitled_XAUI_rx_reset/1
  untitled_XAUI_rx_data/1 -> rx_data/1
  untitled_XAUI_rx_outofband/1 -> rx_outofband/1
  untitled_XAUI_rx_empty/1 -> rx_empty/1
  untitled_XAUI_rx_linkdown/1 -> rx_linkdown/1
  tx_data/1 -> convert_tx_data/1
  convert_tx_data/1 -> untitled_XAUI_tx_data/1
  tx_outofband/1 -> convert_tx_outofband/1
  convert_tx_outofband/1 -> untitled_XAUI_tx_outofband/1
  tx_valid/1 -> convert_tx_valid/1
  convert_tx_valid/1 -> untitled_XAUI_tx_valid/1
  untitled_XAUI_tx_full/1 -> tx_full/1
  untitled_XAUI_tx_data/1 -> Terminator/1
  untitled_XAUI_tx_outofband/1 -> Terminator1/1
  untitled_XAUI_tx_valid/1 -> Terminator2/1
  Constant2/1 -> untitled_XAUI_tx_full/1
  Constant3/1 -> untitled_XAUI_rx_linkdown/1
  Constant4/1 -> untitled_XAUI_rx_empty/1
  Constant5/1 -> untitled_XAUI_rx_outofband/1
  Constant6/1 -> untitled_XAUI_rx_data/1
  untitled_XAUI_rx_get/1 -> Terminator3/1
  untitled_XAUI_rx_reset/1 -> Terminator4/1
  Constant7/1 -> untitled_XAUI_rx_valid/1
  untitled_XAUI_rx_valid/1 -> rx_valid/1
  untitled_XAUI_rx_almost_full/1 -> rx_almost_full/1
  Constant1/1 -> untitled_XAUI_rx_almost_full/1

== system xps_library/XSG core config ==

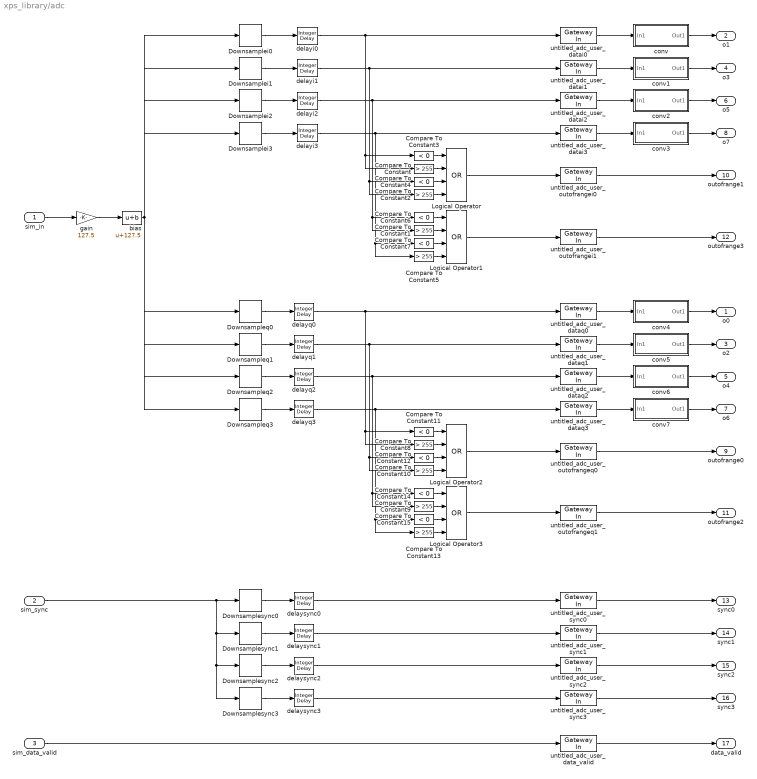
== system xps_library/adc ==
  sim_in : Inport  Port=1  SampleTime=sample_period/8  LatchInput=off
  sim_sync : Inport  Port=2  SampleTime=sample_period/8  LatchInput=off
  sim_data_valid : Inport  Port=3  SampleTime=sample_period/4  LatchInput=off
  Compare To Constant{,1..2,5,8..10,13} (8 alike) : simulink/Logic and Bit Operations/Compare To Constant  relop=>  const=255  LogicOutDataTypeMode=boolean  ZeroCross=off
  Compare To Constant{3..4,6..7,11..12,14..15} (8 alike) : simulink/Logic and Bit Operations/Compare To Constant  relop=<  const=0  LogicOutDataTypeMode=boolean  ZeroCross=off
  Downsamplei0 : dspsigops/Downsample  N=8  phase=1  ic=0  smode=Allow multirate  fmode=Maintain input frame size
  Downsamplei1 : dspsigops/Downsample  N=8  phase=3  ic=0  smode=Allow multirate  fmode=Maintain input frame size
  Downsamplei2 : dspsigops/Downsample  N=8  phase=5  ic=0  smode=Allow multirate  fmode=Maintain input frame size
  Downsamplei3 : dspsigops/Downsample  N=8  phase=7  ic=0  smode=Allow multirate  fmode=Maintain input frame size
  Downsampleq0 : dspsigops/Downsample  N=8  phase=0  ic=0  smode=Allow multirate  fmode=Maintain input frame size
  Downsampleq1 : dspsigops/Downsample  N=8  phase=2  ic=0  smode=Allow multirate  fmode=Maintain input frame size
  Downsampleq2 : dspsigops/Downsample  N=8  phase=4  ic=0  smode=Allow multirate  fmode=Maintain input frame size
  Downsampleq3 : dspsigops/Downsample  N=8  phase=6  ic=0  smode=Allow multirate  fmode=Maintain input frame size
  Downsamplesync0 : dspsigops/Downsample  N=8  phase=0  ic=0  smode=Allow multirate  fmode=Maintain input frame size
  Downsamplesync1 : dspsigops/Downsample  N=8  phase=2  ic=0  smode=Allow multirate  fmode=Maintain input frame size
  Downsamplesync2 : dspsigops/Downsample  N=8  phase=4  ic=0  smode=Allow multirate  fmode=Maintain input frame size
  Downsamplesync3 : dspsigops/Downsample  N=8  phase=6  ic=0  smode=Allow multirate  fmode=Maintain input frame size
  Logical Operator{,1..3} (4 alike) : Logic  Operator=OR  Inputs=4  AllPortsSameDT=off  OutDataTypeMode=Boolean
  bias : Bias  Bias=127.5  SaturateOnIntegerOverflow=on
  conv : Subsystem
  conv1 : Subsystem
  conv2 : Subsystem
  conv3 : Subsystem
  conv4 : Subsystem
  conv5 : Subsystem
  conv6 : Subsystem
  conv7 : Subsystem
  delayi{0..3} (4 alike) : simulink/Discrete/Integer Delay  vinit=0.0  samptime=-1  NumDelays=1
  delayq0 : simulink/Discrete/Integer Delay  vinit=0.0  samptime=-1  NumDelays=2
  delayq1 : simulink/Discrete/Integer Delay  vinit=0.0  samptime=-1  NumDelays=1
  delayq2 : simulink/Discrete/Integer Delay  vinit=0.0  samptime=-1  NumDelays=1
  delayq3 : simulink/Discrete/Integer Delay  vinit=0.0  samptime=-1  NumDelays=1
  delaysync0 : simulink/Discrete/Integer Delay  vinit=0.0  samptime=-1  NumDelays=2
  delaysync1 : simulink/Discrete/Integer Delay  vinit=0.0  samptime=-1  NumDelays=1
  delaysync2 : simulink/Discrete/Integer Delay  vinit=0.0  samptime=-1  NumDelays=1
  delaysync3 : simulink/Discrete/Integer Delay  vinit=0.0  samptime=-1  NumDelays=1
  gain : Gain  Gain=127.5  SaturateOnIntegerOverflow=on
  untitled_adc_user_data_valid : xbsIndex_r3/Gateway In  arith_type=Boolean  n_bits=8  bin_pt=0  quantization="Round  (unbiased: +/- Inf)"  overflow=Saturate  period=sample_period  timing_constraint=None  locs_specified=off  LOCs={}  needs_fixed_name=off  dbl_ovrd=off  show_param=off
      settings: xl_area=[0 0 0 0 8 0 0]
  untitled_adc_user_datai{0..3} (4 alike) : xbsIndex_r3/Gateway In  arith_type=Unsigned  n_bits=8  bin_pt=0  quantization="Round  (unbiased: +/- Inf)"  overflow=Saturate  period=sample_period  timing_constraint=None  locs_specified=off  LOCs={}  needs_fixed_name=off  dbl_ovrd=off  show_param=off
      settings: xl_area=[0 0 0 0 8 0 0]
  untitled_adc_user_dataq{0..3} (4 alike) : xbsIndex_r3/Gateway In  arith_type=Unsigned  n_bits=8  bin_pt=0  quantization="Round  (unbiased: +/- Inf)"  overflow=Saturate  period=sample_period  timing_constraint=None  locs_specified=off  LOCs={}  needs_fixed_name=off  dbl_ovrd=off  show_param=off
      settings: xl_area=[0 0 0 0 8 0 0]
  untitled_adc_user_outofrangei0 : xbsIndex_r3/Gateway In  arith_type=Boolean  n_bits=8  bin_pt=0  quantization="Round  (unbiased: +/- Inf)"  overflow=Saturate  period=sample_period  timing_constraint=None  locs_specified=off  LOCs={}  needs_fixed_name=off  dbl_ovrd=off  show_param=off
      settings: xl_area=[0 0 0 0 8 0 0]
  untitled_adc_user_outofrangei1 : xbsIndex_r3/Gateway In  arith_type=Boolean  n_bits=8  bin_pt=0  quantization="Round  (unbiased: +/- Inf)"  overflow=Saturate  period=sample_period  timing_constraint=None  locs_specified=off  LOCs={}  needs_fixed_name=off  dbl_ovrd=off  show_param=off
      settings: xl_area=[0 0 0 0 8 0 0]
  untitled_adc_user_outofrangeq0 : xbsIndex_r3/Gateway In  arith_type=Boolean  n_bits=8  bin_pt=0  quantization="Round  (unbiased: +/- Inf)"  overflow=Saturate  period=sample_period  timing_constraint=None  locs_specified=off  LOCs={}  needs_fixed_name=off  dbl_ovrd=off  show_param=off
      settings: xl_area=[0 0 0 0 8 0 0]
  untitled_adc_user_outofrangeq1 : xbsIndex_r3/Gateway In  arith_type=Boolean  n_bits=8  bin_pt=0  quantization="Round  (unbiased: +/- Inf)"  overflow=Saturate  period=sample_period  timing_constraint=None  locs_specified=off  LOCs={}  needs_fixed_name=off  dbl_ovrd=off  show_param=off
      settings: xl_area=[0 0 0 0 8 0 0]
  untitled_adc_user_sync{0..3} (4 alike) : xbsIndex_r3/Gateway In  arith_type=Boolean  n_bits=8  bin_pt=0  quantization="Round  (unbiased: +/- Inf)"  overflow=Saturate  period=sample_period  timing_constraint=None  locs_specified=off  LOCs={}  needs_fixed_name=off  dbl_ovrd=off  show_param=off
      settings: xl_area=[0 0 0 0 8 0 0]
  o0 : Outport
  o1 : Outport  Port=2
  o2 : Outport  Port=3
  o3 : Outport  Port=4
  o4 : Outport  Port=5
  o5 : Outport  Port=6
  o6 : Outport  Port=7
  o7 : Outport  Port=8
  outofrange0 : Outport  Port=9
  outofrange1 : Outport  Port=10
  outofrange2 : Outport  Port=11
  outofrange3 : Outport  Port=12
  sync0 : Outport  Port=13
  sync1 : Outport  Port=14
  sync2 : Outport  Port=15
  sync3 : Outport  Port=16
  data_valid : Outport  Port=17
  wires:
  delaysync1/1 -> untitled_adc_user_sync1/1
  delayq3/1 -> untitled_adc_user_dataq3/1, Compare To Constant15/1, Compare To Constant13/1
  delayq2/1 -> untitled_adc_user_dataq2/1, Compare To Constant14/1, Compare To Constant9/1
  delayq1/1 -> untitled_adc_user_dataq1/1, Compare To Constant12/1, Compare To Constant10/1
  delayi3/1 -> untitled_adc_user_datai3/1, Compare To Constant7/1, Compare To Constant5/1
  delayi2/1 -> untitled_adc_user_datai2/1, Compare To Constant6/1, Compare To Constant1/1
  delayi1/1 -> untitled_adc_user_datai1/1, Compare To Constant2/1, Compare To Constant4/1
  Downsamplei0/1 -> delayi0/1
  conv7/1(Out1) -> o6/1
  untitled_adc_user_dataq3/1 -> conv7/1(In1)
  conv6/1(Out1) -> o4/1
  untitled_adc_user_dataq2/1 -> conv6/1(In1)
  conv5/1(Out1) -> o2/1
  untitled_adc_user_dataq1/1 -> conv5/1(In1)
  conv4/1(Out1) -> o0/1
  untitled_adc_user_dataq0/1 -> conv4/1(In1)
  conv3/1(Out1) -> o7/1
  conv2/1(Out1) -> o5/1
  conv1/1(Out1) -> o3/1
  conv/1(Out1) -> o1/1
  untitled_adc_user_sync0/1 -> sync0/1
  untitled_adc_user_outofrangei0/1 -> outofrange1/1
  untitled_adc_user_datai3/1 -> conv3/1(In1)
  untitled_adc_user_datai2/1 -> conv2/1(In1)
  untitled_adc_user_datai1/1 -> conv1/1(In1)
  Downsampleq3/1 -> delayq3/1
  Downsampleq2/1 -> delayq2/1
  Downsampleq1/1 -> delayq1/1
  Downsamplei3/1 -> delayi3/1
  Downsamplei2/1 -> delayi2/1
  Downsamplei1/1 -> delayi1/1
  delayi0/1 -> untitled_adc_user_datai0/1, Compare To Constant/1, Compare To Constant3/1
  Downsampleq0/1 -> delayq0/1
  delayq0/1 -> untitled_adc_user_dataq0/1, Compare To Constant11/1, Compare To Constant8/1
  untitled_adc_user_outofrangei1/1 -> outofrange3/1
  Compare To Constant3/1 -> Logical Operator/1
  Compare To Constant/1 -> Logical Operator/2
  Compare To Constant4/1 -> Logical Operator/3
  Compare To Constant2/1 -> Logical Operator/4
  Logical Operator/1 -> untitled_adc_user_outofrangei0/1
  Compare To Constant6/1 -> Logical Operator1/1
  Compare To Constant1/1 -> Logical Operator1/2
  Compare To Constant7/1 -> Logical Operator1/3
  Compare To Constant5/1 -> Logical Operator1/4
  Logical Operator1/1 -> untitled_adc_user_outofrangei1/1
  untitled_adc_user_outofrangeq0/1 -> outofrange0/1
  untitled_adc_user_outofrangeq1/1 -> outofrange2/1
  Compare To Constant11/1 -> Logical Operator2/1
  Compare To Constant8/1 -> Logical Operator2/2
  Compare To Constant12/1 -> Logical Operator2/3
  Compare To Constant10/1 -> Logical Operator2/4
  Logical Operator2/1 -> untitled_adc_user_outofrangeq0/1
  Compare To Constant14/1 -> Logical Operator3/1
  Compare To Constant9/1 -> Logical Operator3/2
  Compare To Constant15/1 -> Logical Operator3/3
  Compare To Constant13/1 -> Logical Operator3/4
  Logical Operator3/1 -> untitled_adc_user_outofrangeq1/1
  sim_sync/1 -> Downsamplesync0/1, Downsamplesync1/1, Downsamplesync2/1, Downsamplesync3/1
  Downsamplesync0/1 -> delaysync0/1
  Downsamplesync1/1 -> delaysync1/1
  delaysync0/1 -> untitled_adc_user_sync0/1
  untitled_adc_user_sync1/1 -> sync1/1
  Downsamplesync2/1 -> delaysync2/1
  Downsamplesync3/1 -> delaysync3/1
  delaysync2/1 -> untitled_adc_user_sync2/1
  delaysync3/1 -> untitled_adc_user_sync3/1
  untitled_adc_user_sync2/1 -> sync2/1
  untitled_adc_user_sync3/1 -> sync3/1
  untitled_adc_user_data_valid/1 -> data_valid/1
  sim_data_valid/1 -> untitled_adc_user_data_valid/1
  untitled_adc_user_datai0/1 -> conv/1(In1)
  sim_in/1 -> gain/1
  gain/1 -> bias/1
  bias/1 -> Downsamplei0/1, Downsamplei1/1, Downsamplei2/1, Downsamplei3/1, Downsampleq0/1, Downsampleq1/1, Downsampleq2/1, Downsampleq3/1

== system xps_library/corr_adc ==
  sim_din : Inport  Port=1  LatchInput=off
  xps_library_corr_adc_din : S-Function  AncestorBlock=xbsIndex_r3/Gateway In  FunctionName=xlgatewayin  Parameters="arith_type, n_bits, bin_pt, quantization, overflow,  gcb, period, dbl_ovrd, locs_specified, LOCs, timing_constraint, simulinkPeriod, designRoot, 0"  mask(Xilinx Gateway In){arith_type=Unsigned, n_bits=12, bin_pt=data_bin_pt, quantization=Truncate, overflow=Wrap, period=sample_period, timing_constraint=None, locs_specified=off, LOCs={}, needs_fixed_name=off, dbl_ovrd=off, show_param=off, xl_area=[0, 0, 0, 0, 0, 0, 0], xl_use_area=off}
      mask prompts: arith_type "Output Data Type"; n_bits "Number of Bits"; bin_pt "Binary Point"; period "Sample Period"; timing_constraint "IOB Timing Constraint"; locs_specified "Specify IOB Location Constraints"; LOCs "IOB Pad Locations (specify as cell array {'MSB', ..., 'LSB'})"; needs_fixed_name "Do Not Prepend Hierarchy to Port Name"; dbl_ovrd "Override with Double"; show_param "---------------------- Show Implementation Parameters -----------------------------------------------------------------------------------"; xl_area "FPGA Area [Slices, FFs, BRAMs, LUTs, IOBs, Emb. Mults, TBUFs]"; xl_use_area "Use Area Above For Estimation"
      mask help:
      | Gateway in block.  Converts inputs of type Simulink integer, double and fixed point to  Xilinx fixed point type.
      |
      | Hardware notes:  In hardware these blocks become top level input ports.
      mask init:
      | [designRoot, family, part, speed, package, simulinkPeriod, sysclkPeriod, dbl_ovrd, trimVbit] = xlSysgenSettings(gcb,1,0);
      | trimVbit = 1;
      | [bg,fg] = xlcmap('IO',dbl_ovrd);
      | iPos = get_param(gcb,'Position');
      | iWidth=iPos(3)-iPos(1); iHeight=iPos(4)-iPos(2);
      | iCx=iWidth/2;
      | iCy=iHeight/2;
      | [logoX, logoY] = xlogo(iPos);
      mask Help: eval('xlWeb(xlhtmldoclink(''Gateway In''))');
      mask StyleString: popup(Boolean|Unsigned|Signed  (2's comp)),edit,edit,popup(Truncate|Round  (unbiased: +/- Inf)),popup(Wrap|Saturate|Flag as Error),edit,popup(None|Data Rate|Data Rate;  Set 'FAST' Attribute),checkbox,edit,checkbox,checkbox,checkbox,edit,checkbox
      mask CallbackString: xlgatewayinCallback|||||||xlgatewayinCallback||||xlShowIPCallback||
      mask Display:
      | patch([0 iWidth iWidth 0],[0 0 iHeight iHeight] , bg);
      | patch(logoX,logoY , fg);
      | port_label('input',1,'dbl');
      | port_label('output',1,'fpt');
      | 
      | ;plot([0 0 iWidth iWidth 0], [0 iHeight iHeight 0 0]);
  din : Outport
  wires:
  xps_library_corr_adc_din/1 -> din/1
  sim_din/1 -> xps_library_corr_adc_din/1

== system xps_library/corr_dac ==
  data : Inport  Port=1  LatchInput=off
  sync : Inport  Port=2  LatchInput=off
  convert_data : xbsIndex_r3/Convert  arith_type=Unsigned  n_bits=14  bin_pt=bin_pt  quantization=Truncate  overflow=Wrap  latency=0  explicit_period=off  period=sample_period  dbl_ovrd=off  show_param=off  inserted_by_tool=off  pipeline=off
      settings: xl_area=[0, 0, 0, 0, 0, 0, 0]
  convert_sync : xbsIndex_r3/Convert  arith_type=Unsigned  n_bits=1  bin_pt=0  quantization=Truncate  overflow=Wrap  latency=0  explicit_period=off  period=sample_period  dbl_ovrd=off  show_param=off  inserted_by_tool=off  pipeline=off
      settings: xl_area=[0, 0, 0, 0, 0, 0, 0]
  xps_library_corr_dac_data : xbsIndex_r3/Gateway Out  output_type=Double  nbits=8  bin_pt=6  arith_type=Boolean  quantization=Truncate  overflow=Wrap  hdl_port=on  timing_constraint=None  locs_specified=off  LOCs={}  needs_fixed_name=off  show_param=off
      settings: xl_area=[0, 0, 0, 0, 0, 0, 0]
  xps_library_corr_dac_sync : xbsIndex_r3/Gateway Out  output_type=Double  nbits=8  bin_pt=6  arith_type=Boolean  quantization=Truncate  overflow=Wrap  hdl_port=on  timing_constraint=None  locs_specified=off  LOCs={}  needs_fixed_name=off  show_param=off
      settings: xl_area=[0, 0, 0, 0, 0, 0, 0]
  sim_data : Outport
  sim_sync : Outport  Port=2
  wires:
  data/1 -> convert_data/1
  xps_library_corr_dac_data/1 -> sim_data/1
  sync/1 -> convert_sync/1
  xps_library_corr_dac_sync/1 -> sim_sync/1
  convert_sync/1 -> xps_library_corr_dac_sync/1
  convert_data/1 -> xps_library_corr_dac_data/1
